simulink model "FPGA_IN_THE_LOOP_CFAR"  (R2023a)
settings: Solver=VariableStepAuto  StartTime=0.0  StopTime=Tsim  RelTol=1e-3
libraries: fillib x1
settings Model: Creator=mohamed_niazy  LastModifiedBy=mohamed_niazy

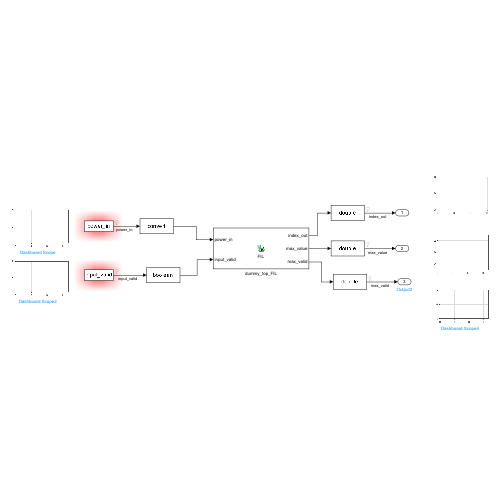
[thumbnail: Simulink's stored preview of the top-level diagram]
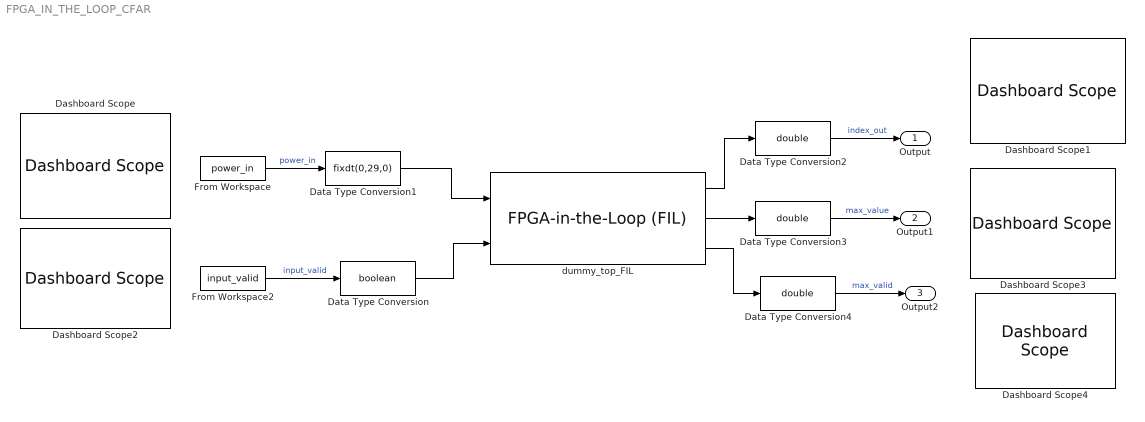
== system FPGA_IN_THE_LOOP_CFAR ==
  Dashboard Scope{,1..4} (5 alike) : DashboardScope
  Data Type Conversion : DataTypeConversion  OutDataTypeStr=boolean  SaturateOnIntegerOverflow=off  RndMeth=Floor
  Data Type Conversion1 : DataTypeConversion  OutDataTypeStr=fixdt(0,29,0)  SaturateOnIntegerOverflow=off  RndMeth=Floor
  Data Type Conversion2 : DataTypeConversion  OutDataTypeStr=double  SaturateOnIntegerOverflow=off  RndMeth=Floor
  Data Type Conversion3 : DataTypeConversion  OutDataTypeStr=double  SaturateOnIntegerOverflow=off  RndMeth=Floor
  Data Type Conversion4 : DataTypeConversion  OutDataTypeStr=double  SaturateOnIntegerOverflow=off  RndMeth=Floor
  From Workspace : FromWorkspace  VariableName=power_in  SampleTime=1
  From Workspace2 : FromWorkspace  VariableName=input_valid  SampleTime=1
  dummy_top_FIL : fillib/FPGA-in-the-Loop (FIL)  ForceInterfaceUpdate=0.12699
  Output : Outport
  Output1 : Outport  Port=2
  Output2 : Outport  Port=3
  wires:
  Data Type Conversion/1 -> dummy_top_FIL/2
  Data Type Conversion1/1 -> dummy_top_FIL/1
  From Workspace/1 -> Data Type Conversion1/1  "power_in"
  From Workspace2/1 -> Data Type Conversion/1  "input_valid"
  dummy_top_FIL/1 -> Data Type Conversion2/1
  dummy_top_FIL/2 -> Data Type Conversion3/1
  dummy_top_FIL/3 -> Data Type Conversion4/1
  Data Type Conversion2/1 -> Output/1  "index_out"
  Data Type Conversion3/1 -> Output1/1  "max_value"
  Data Type Conversion4/1 -> Output2/1  "max_valid"
